simulink library "MotorDriveUnitBasic_utility_lib"  (R2020b)
settings: Solver=VariableStepAuto  StartTime=0.0  StopTime=10.0  RelTol=1e-3
libraries: simulink x2
settings Model: Creator=isaacito  LastModifiedBy=isaacito

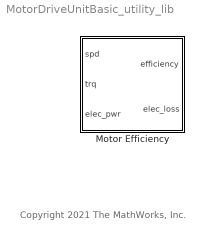
== system MotorDriveUnitBasic_utility_lib ==
  note: Copyright 2021 The MathWorks, Inc.
  Motor Efficiency : Subsystem

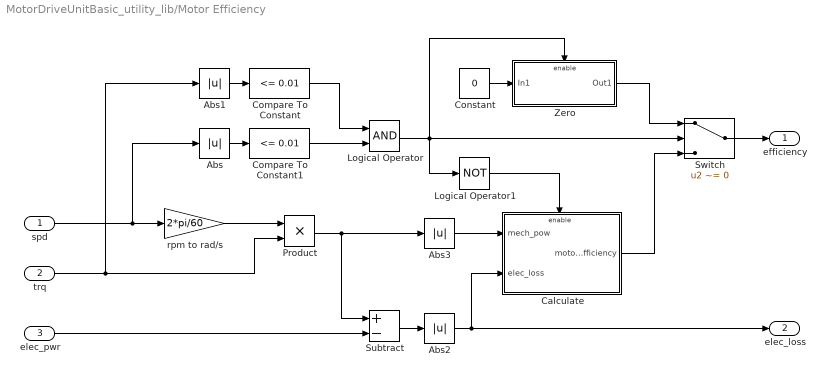
== system MotorDriveUnitBasic_utility_lib/Motor Efficiency ==
  spd : Inport  Unit=rpm
      settings: AttributesFormatString=%<Unit>
  trq : Inport  Port=2  Unit=N*m
      settings: AttributesFormatString=%<Unit>
  elec_pwr : Inport  Port=3  Unit=W
      settings: AttributesFormatString=%<Unit>
  Abs : Abs
  Abs1 : Abs
  Abs2 : Abs  ZeroCross=off
  Abs3 : Abs  ZeroCross=off
  Calculate : Subsystem
  Compare To Constant : simulink/Logic and Bit Operations/Compare To Constant  relop=<=  const=0.01  OutDataTypeStr=boolean
  Compare To Constant1 : simulink/Logic and Bit Operations/Compare To Constant  relop=<=  const=0.01  OutDataTypeStr=boolean
  Constant : Constant  Value=0
  Logical Operator : Logic  AllPortsSameDT=off  OutDataTypeStr=boolean
  Logical Operator1 : Logic  Operator=NOT  AllPortsSameDT=off  OutDataTypeStr=boolean
  Product : Product
  Subtract : Sum  Inputs=+-
  Switch : Switch  Criteria=u2 ~= 0
  Zero : Subsystem  TreatAsAtomicUnit=on
  rpm to rad/s : Gain  Gain=2*pi/60
  efficiency : Outport  Unit=1
      settings: AttributesFormatString=%<Unit>
  elec_loss : Outport  Port=2  Unit=W
      settings: AttributesFormatString=%<Unit>
  wires:
  Abs2/1 -> elec_loss/1, Calculate/2(elec_loss)
  Subtract/1 -> Abs2/1
  elec_pwr/1 -> Subtract/2
  Product/1 -> Abs3/1, Subtract/1
  rpm to rad/s/1 -> Product/1
  Zero/1(Out1) -> Switch/1
  Abs/1 -> Compare To Constant1/1
  Compare To Constant1/1 -> Logical Operator/2
  spd/1 -> rpm to rad/s/1, Abs/1
  Switch/1 -> efficiency/1
  Logical Operator/1 -> Switch/2, Logical Operator1/1, Zero/Enable
  Constant/1 -> Zero/1(In1)
  trq/1 -> Product/2, Abs1/1
  Abs1/1 -> Compare To Constant/1
  Calculate/1(motor efficiency) -> Switch/3
  Logical Operator1/1 -> Calculate/Enable
  Compare To Constant/1 -> Logical Operator/1
  Abs3/1 -> Calculate/1(mech_pow)

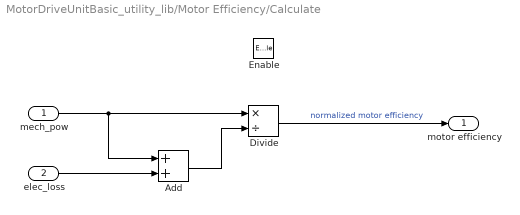
== system MotorDriveUnitBasic_utility_lib/Motor Efficiency/Calculate ==
  mech_pow : Inport  Unit=W
      settings: AttributesFormatString=%<Unit>
  elec_loss : Inport  Port=2  Unit=W
      settings: AttributesFormatString=%<Unit>
  Enable : EnablePort
  Add : Sum
  Divide : Product  Inputs=*/
  motor efficiency : Outport  Unit=1
      settings: AttributesFormatString=%<Unit>
  wires:
  elec_loss/1 -> Add/2
  mech_pow/1 -> Add/1, Divide/1
  Add/1 -> Divide/2
  Divide/1 -> motor efficiency/1  "normalized motor efficiency"

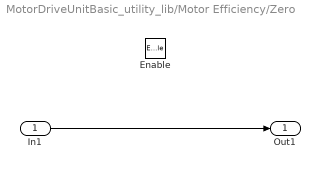
== system MotorDriveUnitBasic_utility_lib/Motor Efficiency/Zero ==
  In1 : Inport
  Enable : EnablePort
  Out1 : Outport
  wires:
  In1/1 -> Out1/1
